simulink model "SimulinkCurvePV"  (R2022b)
settings: Solver=VariableStepAuto  StartTime=0.0  StopTime=1.1  RelTol=1e-3
libraries: spsDiodeLib x11, spsPVArrayLib x10, spsSeriesRLCBranchLib x5, spsControlledVoltageSourceLib x1, spsCurrentMeasurementLib x1, simulink x1, spsVoltageMeasurementLib x1, sps_lib x1
settings Model: Creator=LE QUOC DINH  LastModifiedBy=LE QUOC DINH

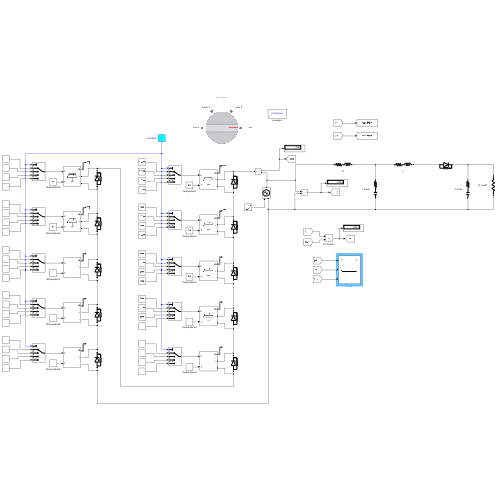
[thumbnail: Simulink's stored preview of the top-level diagram]
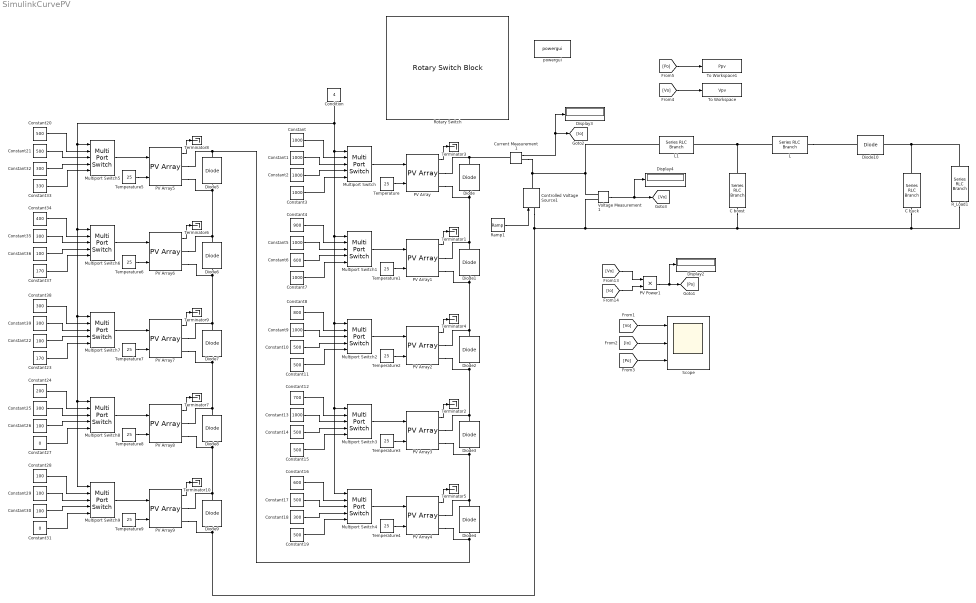
== system SimulinkCurvePV ==
  C boost : spsSeriesRLCBranchLib/Series RLC Branch  LConnTagsString=__new0  RConnTagsString=__new0  BranchType=RC  Resistance=1  Inductance=1e-3  SetiL0=off  InitialCurrent=0  Capacitance=5e-3  Setx0=off  InitialVoltage=0  Measurements=None
  C buck : spsSeriesRLCBranchLib/Series RLC Branch  LConnTagsString=__new0  RConnTagsString=__new0  BranchType=RC  Resistance=1  Inductance=1e-3  SetiL0=off  InitialCurrent=0  Capacitance=5e-6  Setx0=off  InitialVoltage=0  Measurements=None
  Condition : Constant  Value=4
  Constant{,1..3,5,7,9,13} (8 alike) : Constant  Value=1000
  Constant{10..11,14..15,17,19..21} (8 alike) : Constant  Value=500
  Constant12 : Constant  Value=700
  Constant16 : Constant  Value=600
  Constant{18,25,32,35,38..39} (6 alike) : Constant  Value=300
  Constant{22,26,28..30,36} (6 alike) : Constant  Value=100
  Constant23 : Constant  Value=170
  Constant24 : Constant  Value=200
  Constant27 : Constant  Value=0
  Constant31 : Constant  Value=0
  Constant33 : Constant  Value=330
  Constant34 : Constant  Value=400
  Constant37 : Constant  Value=170
  Constant4 : Constant  Value=900
  Constant6 : Constant  Value=600
  Constant8 : Constant  Value=800
  Controlled Voltage Source1 : spsControlledVoltageSourceLib/Controlled Voltage Source  Initialize=on  Source_Type=DC  Amplitude=0  Phase=0  Frequency=0  Measurements=None
  Current Measurement1 : spsCurrentMeasurementLib/Current Measurement  PhasorSimulation=off  OutputType=Complex  PSBequivalent=0
  Diode{,1..10} (11 alike) : spsDiodeLib/Diode  Ron=0.001  Lon=0  Vf=0.8  IC=0  UseSnubber=0  Rs=500  Cs=250e-9  Measurements=off
  Display2 : Display
  Display3 : Display
  Display4 : Display
  L : spsSeriesRLCBranchLib/Series RLC Branch  LConnTagsString=__new0  RConnTagsString=__new0  BranchType=RL  Resistance=1  Inductance=5e-3  SetiL0=off  InitialCurrent=0  Capacitance=1e-6  Setx0=off  InitialVoltage=0  Measurements=None
  L1 : spsSeriesRLCBranchLib/Series RLC Branch  LConnTagsString=__new0  RConnTagsString=__new0  BranchType=RL  Resistance=1  Inductance=5e-3  SetiL0=off  InitialCurrent=0  Capacitance=1e-6  Setx0=off  InitialVoltage=0  Measurements=None
  Multiport Switch{,1..9} (10 alike) : MultiPortSwitch  Inputs=4  SaturateOnIntegerOverflow=off  InputSameDT=off
  PV Array{,1..9} (10 alike) : spsPVArrayLib/PV Array  Npar=1  Nser=1  PlotType=array @ 25 deg.C & specified irradiances  S_vec="[ 1000  500  100 ]"  Temp_C_vec="[ 45 25  ]"  ModuleName=Mitsubishi Electric PV-EE125MF5F  PlotWhenSelected=off  Pm=125.079  Ncell=36  Voc=21.8  Isc=7.9  Vm=17.3  Im=7.23  beta_Voc_pc=-0.3637  alpha_Isc_pc=0.042696  beta_Voc=-0.079287  alpha_Isc=0.003373  IL=7.9305  I0=2.9341e-10  nI=0.98298  Rsh=66.3188  Rs=0.25575  RobustModel=off  RobustCellTemperature=313.3991  BAL=off  Tc=20  Tfilter=0.1
  PV Power1 : Product
  R_Load1 : spsSeriesRLCBranchLib/Series RLC Branch  LConnTagsString=__new0  RConnTagsString=__new0  BranchType=R  Resistance=30  Inductance=50e-6  SetiL0=off  InitialCurrent=0  Capacitance=1000e-6  Setx0=off  InitialVoltage=0  Measurements=None
  Ramp1 : simulink/Sources/Ramp  slope=21.8*10  start=0  InitialOutput=0
  Rotary Switch : RotarySwitchBlock
      settings: Values={{'Condition A', 'Condition B', 'Condition C', 'Condition D'}, [1 2 3 4]}
  Scope : Scope  NumInputPorts=3
  Temperature{,1..9} (10 alike) : Constant  Value=25
  Terminator{1..10} (10 alike) : Terminator
  To Workspace : ToWorkspace  VariableName=Vpv  SaveFormat=Structure With Time  SampleTime=-1
  To Workspace1 : ToWorkspace  VariableName=Ppv  SaveFormat=Structure With Time  SampleTime=-1
  Voltage Measurement1 : spsVoltageMeasurementLib/Voltage Measurement  PhasorSimulation=off  OutputType=Complex  PSBequivalent=0
  powergui : sps_lib/powergui  Priority=1  SimulationMode=Continuous  SampleTime=1e-6  frequency=60  Iterations=50  frequencyindice=0  Pbase=100e6  ErrMax=1e-4  UnitsV=kV  UnitsW=MW  buscounter=0  FunctionMessages=off  echomessages=off  EnableUseOfTLC=off  CurrentSourceSwitches=off  DisableSnubberDevices=off  DisableRonSwitches=off  DisableVfSwitches=off  DisplayEquations=off  AutomaticDiscreteSolvers=off  SolverType=Tustin/Backward Euler (TBE)  Interpol=off  ExternalGateDelay=off  methode=off  Ts=100  x0status=blocks  SPID=on  SwTol=0  HookPort=off  NonlinearTolerance=0  nMaxIteration=15  ContinueOnMaxIteration=off  RestoreLinks=warning  ResistiveCurrentMeasurement=off  Frange=[0:2:500]  Ylog=off  Xlog=on  ShowGrid=off  save=off  variable=ZData  structure=0  ZoomFFT=off  StartTime=0.0  cycles=1  DisplayStyle=1  fundamental=60  FreqAxis=off  MaxFrequency=1000  frequencyindicesteady=1  RmsSteady=1  display=off
  wires:
  Voltage Measurement1/1 -> Display4/1, [Vo]
  PV Array5/1 -> Terminator8/1
  Constant24/1 -> Multiport Switch8/2
  Constant17/1 -> Multiport Switch4/3
  [Po] -> Scope/3
  Constant21/1 -> Multiport Switch5/3
  Constant27/1 -> Multiport Switch8/5
  Constant1/1 -> Multiport Switch/3
  [Vo] -> Scope/1
  [Io] -> Scope/2
  Multiport Switch5/1 -> PV Array5/1
  Constant25/1 -> Multiport Switch8/3
  Constant/1 -> Multiport Switch/2
  Constant35/1 -> Multiport Switch6/3
  PV Array4/1 -> Terminator5/1
  Multiport Switch6/1 -> PV Array6/1
  Constant36/1 -> Multiport Switch6/4
  Constant32/1 -> Multiport Switch5/4
  Constant33/1 -> Multiport Switch5/5
  PV Array6/1 -> Terminator6/1
  Ramp1/1 -> Controlled Voltage Source1/1
  PV Array7/1 -> Terminator9/1
  Constant20/1 -> Multiport Switch5/2
  Constant26/1 -> Multiport Switch8/4
  Constant29/1 -> Multiport Switch9/3
  PV Array8/1 -> Terminator7/1
  Constant13/1 -> Multiport Switch3/3
  Temperature6/1 -> PV Array6/2
  Constant2/1 -> Multiport Switch/4
  Temperature7/1 -> PV Array7/2
  Constant39/1 -> Multiport Switch7/3
  Temperature8/1 -> PV Array8/2
  Multiport Switch/1 -> PV Array/1
  Constant7/1 -> Multiport Switch1/5
  Constant28/1 -> Multiport Switch9/2
  Constant19/1 -> Multiport Switch4/5
  Temperature/1 -> PV Array/2
  Constant30/1 -> Multiport Switch9/4
  Constant14/1 -> Multiport Switch3/4
  Condition/1 -> Multiport Switch5/1, Multiport Switch6/1, Multiport Switch8/1, Multiport Switch9/1, Multiport Switch7/1, Multiport Switch2/1, Multiport Switch4/1, Multiport Switch3/1, Multiport Switch1/1, Multiport Switch/1
  Constant38/1 -> Multiport Switch7/2
  Constant4/1 -> Multiport Switch1/2
  PV Array1/1 -> Terminator1/1
  Constant31/1 -> Multiport Switch9/5
  Temperature4/1 -> PV Array4/2
  Temperature9/1 -> PV Array9/2
  Constant16/1 -> Multiport Switch4/2
  Multiport Switch7/1 -> PV Array7/1
  Multiport Switch9/1 -> PV Array9/1
  PV Array9/1 -> Terminator10/1
  Constant22/1 -> Multiport Switch7/4
  Multiport Switch2/1 -> PV Array2/1
  PV Array2/1 -> Terminator4/1
  Constant10/1 -> Multiport Switch2/4
  Constant23/1 -> Multiport Switch7/5
  Temperature2/1 -> PV Array2/2
  Constant8/1 -> Multiport Switch2/2
  Constant11/1 -> Multiport Switch2/5
  Current Measurement1/1 -> [Io], Display3/1
  Constant34/1 -> Multiport Switch6/2
  Constant12/1 -> Multiport Switch3/2
  Constant9/1 -> Multiport Switch2/3
  PV Power1/1 -> [Po], Display2/1
  Temperature5/1 -> PV Array5/2
  Multiport Switch4/1 -> PV Array4/1
  PV Array3/1 -> Terminator2/1
  Temperature1/1 -> PV Array1/2
  Constant18/1 -> Multiport Switch4/4
  Temperature3/1 -> PV Array3/2
  [Vo] -> PV Power1/1
  Constant37/1 -> Multiport Switch6/5
  Multiport Switch3/1 -> PV Array3/1
  Multiport Switch1/1 -> PV Array1/1
  Constant3/1 -> Multiport Switch/5
  [Io] -> PV Power1/2
  Constant15/1 -> Multiport Switch3/5
  Constant6/1 -> Multiport Switch1/4
  PV Array/1 -> Terminator3/1
  Constant5/1 -> Multiport Switch1/3
  Multiport Switch8/1 -> PV Array8/1
  [Po] -> To Workspace1/1
  [Vo] -> To Workspace/1
  connections:
  Diode1/RConn1 -- PV Array1/RConn1 -- PV Array/RConn2 -- Diode/LConn1
  Current Measurement1/RConn1 -- L1/LConn1 -- Voltage Measurement1/LConn1 -- Controlled Voltage Source1/RConn1
  C buck/LConn1 -- R_Load1/LConn1 -- Diode10/RConn1
  C boost/LConn1 -- L1/RConn1 -- L/LConn1
  C buck/RConn1 -- C boost/RConn1 -- Voltage Measurement1/LConn2 -- Controlled Voltage Source1/LConn1 -- Diode9/LConn1 -- PV Array9/RConn2 -- R_Load1/RConn1
  PV Array8/RConn1 -- Diode7/LConn1 -- PV Array7/RConn2 -- Diode8/RConn1
  PV Array7/RConn1 -- PV Array6/RConn2 -- Diode6/LConn1 -- Diode7/RConn1
  PV Array6/RConn1 -- Diode6/RConn1 -- PV Array5/RConn2 -- Diode5/LConn1
  PV Array9/RConn1 -- Diode8/LConn1 -- PV Array8/RConn2 -- Diode9/RConn1
  PV Array4/RConn1 -- Diode4/RConn1 -- Diode3/LConn1 -- PV Array3/RConn2
  Diode3/RConn1 -- PV Array3/RConn1 -- PV Array2/RConn2 -- Diode2/LConn1
  Diode4/LConn1 -- PV Array5/RConn1 -- Diode5/RConn1 -- PV Array4/RConn2
  Diode1/LConn1 -- PV Array2/RConn1 -- Diode2/RConn1 -- PV Array1/RConn2
  Diode/RConn1 -- PV Array/RConn1 -- Current Measurement1/LConn1
  L/RConn1 -- Diode10/LConn1
